simulink model "UAV_USV_Simulator"  (R2017b)
settings: Solver=ode3  StartTime=0.0  StopTime=15  FixedStep=0.01  RelTol=1e-3
PreLoadFcn:
  | addpath(genpath(fileparts(which (bdroot))))
  | 
  | CascadedPID=Simulink.Variant('ControlType==0');
  | InverseKin=Simulink.Variant('ControlType==1');
  | 
  | ControlType = 0;
  | Waypoints = [10 10 ; -10 10 ; -10 -10; 10 -10; 0 0 ];
  | WaypointsX = Waypoints(:,1)'/3;
  | WaypointsY = Waypoints(:,2)'/3;
  | StriderSpeedCmd = 0;
  | 
  | ax=0;
  | ay=0;
  | LandingSchedule = 5;
  | EnableVTOL=1;
  | Psi_cmd = 0;
  | Alt_cmd = 1;
  | 
  | AccRadius =0.5;
  | AppAlt =1;
  | e = 0.1;
PostLoadFcn:
  | addpath(genpath(fileparts(which (bdroot))))
model workspace (MAT data in the model file):
  CD = Simulink.Parameter
  CD.Value = 2.38e-07
  CD.Description = 'Drag/Torque coefficient for the quadcopter rotors'
  CD.DataType = 'auto'
  CD.Dimensions = [1 1]
  CT = Simulink.Parameter
  CT.Value = 9.148e-06
  CT.Description = 'Thrust coefficient for the quadcopter rotors'
  CT.DataType = 'auto'
  CT.Dimensions = [1 1]
  MaxRPM = Simulink.Parameter
  MaxRPM.Value = 5000
  MaxRPM.DataType = 'auto'
  MaxRPM.Dimensions = [1 1]
  RPM2RAD = Simulink.Parameter
  RPM2RAD.Value = 0.10471975512
  RPM2RAD.DataType = 'auto'
  RPM2RAD.Dimensions = [1 1]
  g = Simulink.Parameter
  g.Value = 9.81
  g.DataType = 'auto'
  g.Dimensions = [1 1]
  mass = Simulink.Parameter
  mass.Value = 0.441
  mass.Description = 'Mass of the quadcopter'
  mass.DataType = 'auto'
  mass.Dimensions = [1 1]
undefined symbols (not defined in the file or in its folder): magnitude, sigbuilder_block
libraries: simulink x12, simulink_extras x12, vrlib x5, dsparch4 x1, sharedtransform x1, dspswit3 x1
(part 1 of 2)
settings Model: Creator=Omar Velasco Anrar  LastModifiedBy=omarc
settings DataIOCC: ReturnWorkspaceOutputs=on
settings OptimizationCC: EfficientMapNaN2IntZero=off
settings DebuggingCC: ReadBeforeWriteMsg=DisableAll  WriteAfterWriteMsg=DisableAll  WriteAfterReadMsg=DisableAll  MultiTaskDSMMsg=none
settings HardwareCC: TargetBitPerPointer=64  TargetBitPerSizeT=64  TargetBitPerPtrDiffT=64  TargetLongLongMode=on  TargetIntDivRoundTo=Zero  TargetEndianess=LittleEndian  TargetWordSize=64  TargetHWDeviceType=MATLAB Host  ProdEqTarget=off
settings ModelReferenceCC: UpdateModelReferenceTargets=IfOutOfDate
settings SFSimCC: SFSimEcho=off
settings CodeAppCC: MaxIdLength=128
settings GRTTargetCC: TargetLangStandard=C89/C90 (ANSI)  CombineOutputUpdateFcns=off  GRTInterface=on

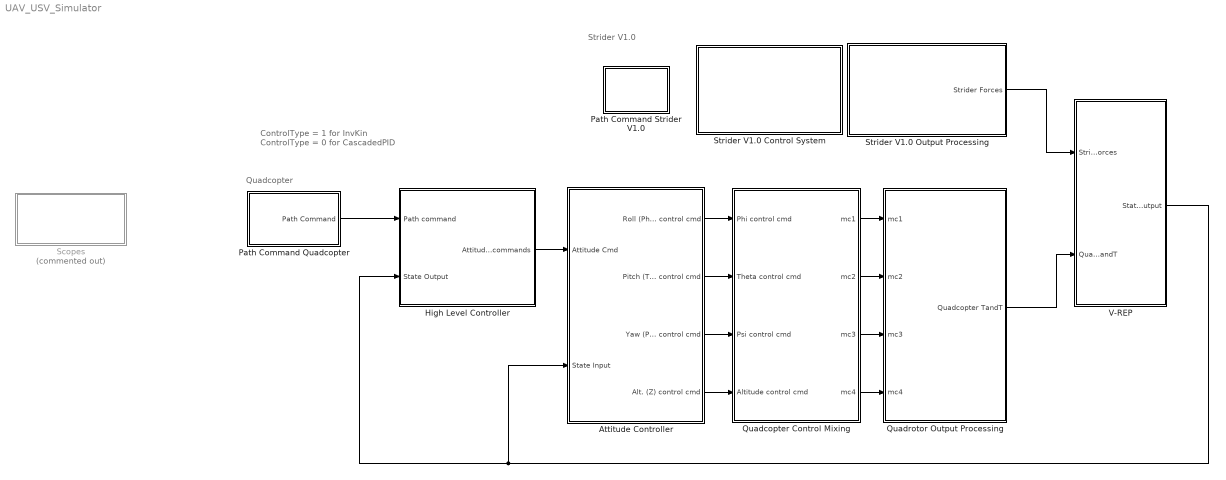
== system UAV_USV_Simulator ==
  note: Quadcopter
  note: Strider V1.0
  note: ControlType = 1 for InvKin
      | ControlType = 0 for CascadedPID
  Attitude Controller : Subsystem
  High Level Controller : Subsystem  Variant=on
  Path Command Quadcopter : Subsystem  Variant=on
  Path Command Strider V1.0 : Subsystem
  Quadcopter Control Mixing : Subsystem
  Quadrotor Output Processing : Subsystem
  "Scopes " : Subsystem  Commented=on
  Strider V1.0 Output Processing : Subsystem
  Strider V1.0 Control System : Subsystem
  V-REP : Subsystem
  wires:
  Quadcopter Control Mixing/4(mc4) -> Quadrotor Output Processing/4(mc4)
  V-REP/1(State Output) -> High Level Controller/2(State Output), Attitude Controller/2(State Input)
  Attitude Controller/4(Alt. (Z) control cmd) -> Quadcopter Control Mixing/4(Altitude control cmd)
  Attitude Controller/2(Pitch (Theta) control cmd) -> Quadcopter Control Mixing/2(Theta control cmd)
  Attitude Controller/3(Yaw (Psi) control cmd) -> Quadcopter Control Mixing/3(Psi control cmd)
  Quadcopter Control Mixing/2(mc2) -> Quadrotor Output Processing/2(mc2)
  Quadcopter Control Mixing/3(mc3) -> Quadrotor Output Processing/3(mc3)
  Quadcopter Control Mixing/1(mc1) -> Quadrotor Output Processing/1(mc1)
  Attitude Controller/1(Roll (Phi) control cmd) -> Quadcopter Control Mixing/1(Phi control cmd)
  High Level Controller/1(Attitude commands) -> Attitude Controller/1(Attitude Cmd)
  Path Command Quadcopter/1(Path Command) -> High Level Controller/1(Path command)
  Quadrotor Output Processing/1("Quadcopter TandT ") -> V-REP/2(Quadcopter TandT)
  Strider V1.0 Output Processing/1(Strider Forces) -> V-REP/1(Strider Forces)

== system UAV_USV_Simulator/Attitude Controller ==
  Attitude Cmd : Inport
  State Input : Inport  Port=2
  Altitude Control : Subsystem
  Bus Selector : BusSelector  OutputSignals=Phi,The,Psi,Z
  Pitch Control : Subsystem
  Roll Control : Subsystem
  Yaw Control : Subsystem
  Roll (Phi) control cmd : Outport
  Pitch (Theta) control cmd : Outport  Port=2
  Yaw (Psi) control cmd : Outport  Port=3
  Alt. (Z) control cmd : Outport  Port=4
  tag scope: Cmds=global
  wires:
  State Input/1 -> Bus Selector/1
  Bus Selector/1 -> Roll Control/2(Phi)  "<Phi>"
  Bus Selector/2 -> Pitch Control/2(Theta)  "<The>"
  Bus Selector/3 -> Yaw Control/2(Psi)  "<Psi>"
  Yaw Control/1(Out1) -> Yaw (Psi) control cmd/1
  Pitch Control/1(Out1) -> Pitch (Theta) control cmd/1
  Roll Control/1(Out1) -> Roll (Phi) control cmd/1
  Attitude Cmd/1 -> Altitude Control/1("Alt_cmd "), Yaw Control/1(Attitude Comand), Pitch Control/1(Attitude Comand), Roll Control/1(Attitude Comand), [Cmds]
  Altitude Control/1(Out) -> Alt. (Z) control cmd/1
  Bus Selector/4 -> Altitude Control/2(Z)  "<Z>"

== system UAV_USV_Simulator/High Level Controller ==
  Path command : Inport
  State Output : Inport  Port=2
  Cascaded PID : Subsystem  VariantControl=CascadedPID
  Inverse kinematics architecture : Subsystem  VariantControl=InverseKin
  Attitude commands : Outport

== system UAV_USV_Simulator/Path Command Quadcopter ==
  "Cascaded PID " : Subsystem  VariantControl=CascadedPID
  Inverse Kinematics : Subsystem  VariantControl=InverseKin
  Path Command : Outport

== system UAV_USV_Simulator/Path Command Strider V1.0 ==
  Constant : Constant  Value=WaypointsX
  Constant1 : Constant  Value=StriderSpeedCmd
  Constant2 : Constant  Value=WaypointsY
  Gain : Gain
  Gain1 : Gain
  tag scope: Speed_command=global, X_waypoints=global, Y_waypoints=global
  wires:
  Constant1/1 -> [Speed_command]
  Gain/1 -> [Y_waypoints]
  Gain1/1 -> [X_waypoints]
  Constant2/1 -> Gain/1
  Constant/1 -> Gain1/1

== system UAV_USV_Simulator/Quadcopter Control Mixing ==
  Phi control cmd : Inport
  Theta control cmd : Inport  Port=2
  Psi control cmd : Inport  Port=3
  Altitude control cmd : Inport  Port=4
  + Config Control Mixing : Subsystem
  mc1 : Outport
  mc2 : Outport  Port=2
  mc3 : Outport  Port=3
  mc4 : Outport  Port=4
  wires:
  Phi control cmd/1 -> + Config Control Mixing/1(Phi rotor cmd)
  Theta control cmd/1 -> + Config Control Mixing/2(Theta rotor cmd)
  Psi control cmd/1 -> + Config Control Mixing/3(Psi rotor cmd)
  Altitude control cmd/1 -> + Config Control Mixing/4(Altitude rotor cmd)
  + Config Control Mixing/1(mc1) -> mc1/1  "mc1"
  + Config Control Mixing/2(mc2) -> mc2/1  "mc2"
  + Config Control Mixing/3(mc3) -> mc3/1  "mc3"
  + Config Control Mixing/4(mc4) -> mc4/1  "mc4"

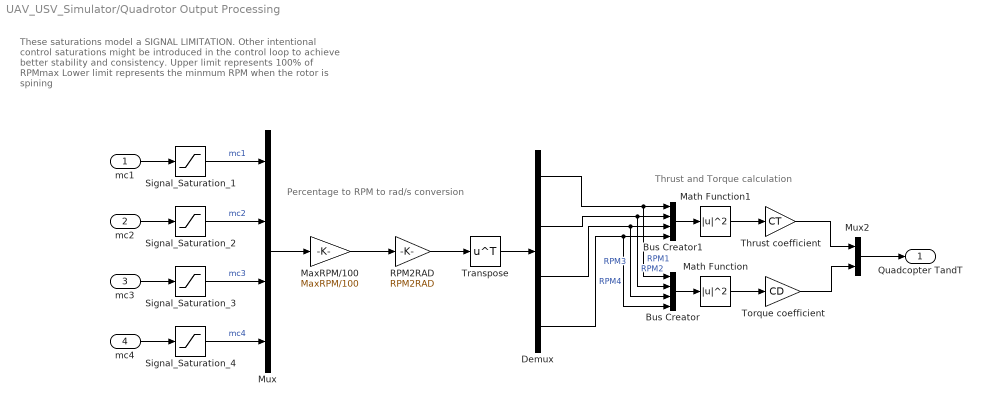
== system UAV_USV_Simulator/Quadrotor Output Processing ==
  note: Percentage to RPM to rad/s conversion
  note: Thrust and Torque calculation
  note: These saturations model a SIGNAL LIMITATION.
      | Other intentional control saturations might be introduced in the
      | control loop to achieve better stability and consistency.
      | Upper limit represents 100% of RPMmax
      | Lower limit represents the minmum RPM when the rotor is spining
  mc1 : Inport
  mc2 : Inport  Port=2
  mc3 : Inport  Port=3
  mc4 : Inport  Port=4
  Bus Creator : BusCreator  Inputs=4
  Bus Creator1 : BusCreator  Inputs=4
  Demux : Demux
  Math Function : Math  Operator=magnitude^2  SaturateOnIntegerOverflow=on
  Math Function1 : Math  Operator=magnitude^2  SaturateOnIntegerOverflow=on
  MaxRPM/100 : Gain  Gain=MaxRPM/100
  Mux : Mux
  Mux2 : Mux  Inputs=2
  RPM2RAD : Gain  Gain=RPM2RAD
  Signal_Saturation_{1..4} (4 alike) : Saturate  UpperLimit=100  LowerLimit=0  ZeroCross=off
  Thrust coefficient : Gain  Gain=CT
  Torque coefficient : Gain  Gain=CD
  Transpose : Math  Operator=transpose  SaturateOnIntegerOverflow=on
  "Quadcopter TandT " : Outport
  wires:
  mc1/1 -> Signal_Saturation_1/1
  mc4/1 -> Signal_Saturation_4/1
  Signal_Saturation_1/1 -> Mux/1  "mc1"
  Signal_Saturation_2/1 -> Mux/2  "mc2"
  Demux/1 -> Bus Creator/1, Bus Creator1/1  "RPM1"
  Demux/2 -> Bus Creator/2, Bus Creator1/2  "RPM2"
  Demux/3 -> Bus Creator/3, Bus Creator1/3  "RPM3"
  Demux/4 -> Bus Creator/4, Bus Creator1/4  "RPM4"
  MaxRPM/100/1 -> RPM2RAD/1
  Mux/1 -> MaxRPM/100/1
  Signal_Saturation_4/1 -> Mux/4  "mc4"
  Bus Creator/1 -> Math Function/1
  Torque coefficient/1 -> Mux2/2
  Thrust coefficient/1 -> Mux2/1
  Math Function/1 -> Torque coefficient/1
  Bus Creator1/1 -> Math Function1/1
  Math Function1/1 -> Thrust coefficient/1
  RPM2RAD/1 -> Transpose/1
  Transpose/1 -> Demux/1
  mc2/1 -> Signal_Saturation_2/1
  mc3/1 -> Signal_Saturation_3/1
  Signal_Saturation_3/1 -> Mux/3  "mc3"
  Mux2/1 -> "Quadcopter TandT "/1

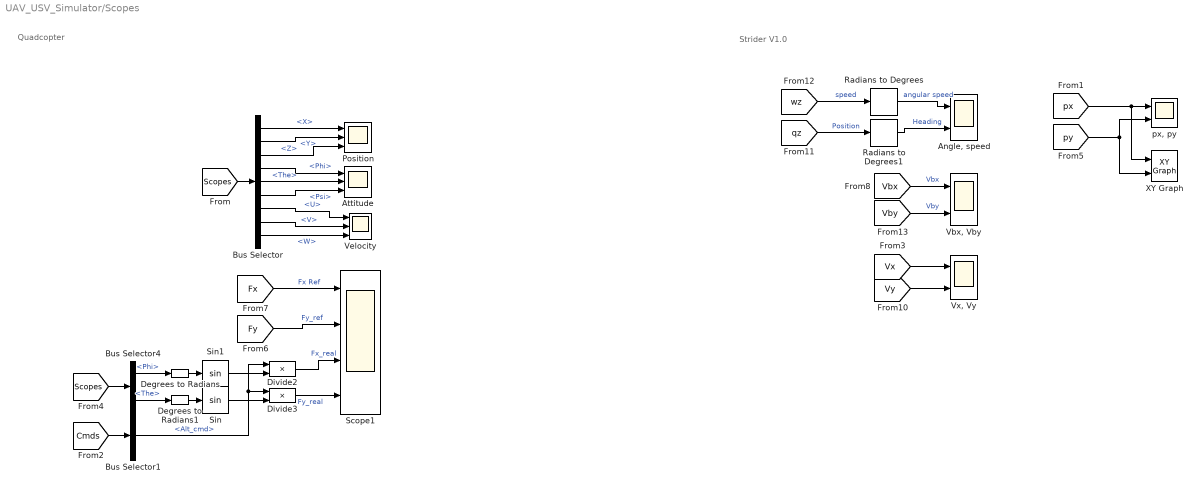
== system UAV_USV_Simulator/Scopes  ==
  note: Strider V1.0
  note: Quadcopter
  "Angle, speed" : Scope  NumInputPorts=2
  Attitude : Scope  NumInputPorts=3
  Bus Selector : BusSelector  OutputSignals=X,Y,Z,Phi,The,Psi,U,V,W
  Bus Selector1 : BusSelector  OutputSignals=Alt_cmd
  Bus Selector4 : BusSelector  OutputSignals=Phi,The
  Degrees to Radians : simulink_extras/Transformations/Degrees to Radians
  Degrees to Radians1 : simulink_extras/Transformations/Degrees to Radians
  Divide2 : Product  Inputs=**
  Divide3 : Product  Inputs=**
  Position : Scope  NumInputPorts=3
  Radians to Degrees : simulink_extras/Transformations/Radians to Degrees
  Radians to Degrees1 : simulink_extras/Transformations/Radians to Degrees
  Scope1 : Scope  NumInputPorts=4
  Sin : Trigonometry
  Sin1 : Trigonometry
  "Vbx, Vby" : Scope  NumInputPorts=2
  Velocity : Scope  NumInputPorts=3
  "Vx, Vy" : Scope  NumInputPorts=2
  XY Graph : simulink/Sinks/XY Graph  xmin=-15  xmax=15  ymin=-15  ymax=15  st=-1
  "px, py" : Scope  NumInputPorts=2
  wires:
  Bus Selector4/1 -> Degrees to Radians/1  "<Phi>"
  Bus Selector4/2 -> Degrees to Radians1/1  "<The>"
  Sin1/1 -> Divide2/2
  [Fy] -> Scope1/2  "Fy_ref"
  [Fx] -> Scope1/1  "Fx Ref"
  Sin/1 -> Divide3/2
  Divide3/1 -> Scope1/4  "Fy_real"
  Divide2/1 -> Scope1/3  "Fx_real"
  Degrees to Radians/1 -> Sin1/1
  Degrees to Radians1/1 -> Sin/1
  [Scopes] -> Bus Selector4/1
  ? -> ?
  Bus Selector/6 -> Attitude/3  "<Psi>"
  Bus Selector/9 -> Velocity/3  "<W>"
  Bus Selector/4 -> Attitude/1  "<Phi>"
  Bus Selector/7 -> Velocity/1  "<U>"
  [Scopes] -> Bus Selector/1
  Bus Selector/5 -> Attitude/2  "<The>"
  Bus Selector/8 -> Velocity/2  "<V>"
  Bus Selector/2 -> Position/2  "<Y>"
  Bus Selector/3 -> Position/3  "<Z>"
  Bus Selector/1 -> Position/1  "<X>"
  [Vx] -> "Vx, Vy"/1
  [Vbx] -> "Vbx, Vby"/1  "Vbx"
  [wz] -> Radians to Degrees/1  "speed"
  [qz] -> Radians to Degrees1/1  "Position"
  Radians to Degrees1/1 -> "Angle, speed"/2  "Heading"
  [Vby] -> "Vbx, Vby"/2  "Vby"
  Radians to Degrees/1 -> "Angle, speed"/1  "angular speed"
  [Vy] -> "Vx, Vy"/2
  [py] -> XY Graph/2, "px, py"/2
  [px] -> XY Graph/1, "px, py"/1
  [Cmds] -> Bus Selector1/1
  Bus Selector1/1 -> Divide3/1, Divide2/1  "<Alt_cmd>"

== system UAV_USV_Simulator/Strider V1.0 Output Processing ==
  Friction forces : Subsystem
  Hydrodinamic forces : Subsystem
  "Inertial to body frame speed " : Subsystem
  Mux3 : Mux  Inputs=6
  Rudder forces1 : Subsystem
  Sum1 : Sum  Inputs=|++
  Strider Forces : Outport
  wires:
  Rudder forces1/2(Y rudder force) -> Mux3/3
  [Thrust_cmd] -> Mux3/1
  Rudder forces1/1(X rudder force) -> Mux3/2
  Mux3/1 -> Strider Forces/1
  Friction forces/2(Ff Y) -> Sum1/1
  Hydrodinamic forces/1(Yhyd) -> Sum1/2
  Friction forces/1(Ff X) -> Mux3/4
  Sum1/1 -> Mux3/5
  Hydrodinamic forces/2(Nhyd) -> Mux3/6

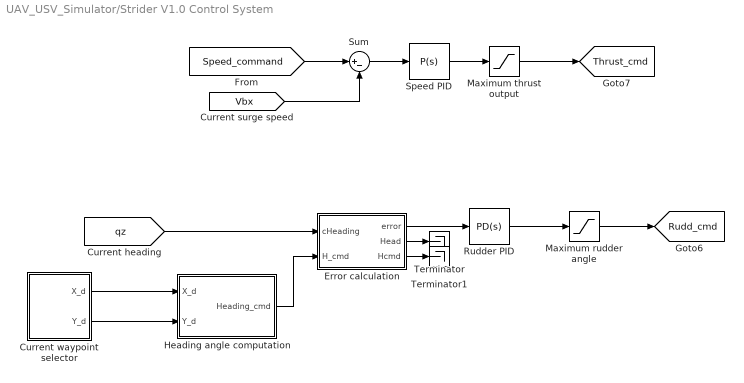
== system UAV_USV_Simulator/Strider V1.0 Control System ==
  Current waypoint selector : Subsystem
  Error calculation : MATLAB Function  TreatAsAtomicUnit=on
  Heading angle computation : Subsystem
  Maximum rudder angle : Saturate  UpperLimit=35*pi/180  LowerLimit=-35*pi/180
  Maximum thrust output : Saturate  UpperLimit=3  LowerLimit=-3
  Rudder PID : simulink/Continuous/PID Controller  Controller=PD  TimeDomain=Continuous-time  SampleTime=-1  IntegratorMethod=Forward Euler  FilterMethod=Forward Euler  Form=Parallel  UseFilter=on  ControllerParametersSource=internal  P=0.5  I=1  D=0.6  N=21.4165136740303  InitialConditionSource=internal  InitialConditionForIntegrator=0  InitialConditionForFilter=0  ExternalReset=none  LimitOutput=off  UpperSaturationLimit=inf  LowerSaturationLimit=-inf  LinearizeAsGain=on  AntiWindupMode=none  Kb=1  TrackingMode=off  Kt=1  PParamMin=[]  PParamMax=[]  IParamMin=[]  IParamMax=[]  DParamMin=[]  DParamMax=[]  NParamMin=[]  NParamMax=[]  KbParamMin=[]  KbParamMax=[]  KtParamMin=[]  KtParamMax=[]  POutMin=[]  POutMax=[]  IOutMin=[]  IOutMax=[]  DOutMin=[]  DOutMax=[]  NOutMin=[]  NOutMax=[]  KbOutMin=[]  KbOutMax=[]  KtOutMin=[]  KtOutMax=[]  IntegratorOutMin=[]  IntegratorOutMax=[]  FilterOutMin=[]  FilterOutMax=[]  SumOutMin=[]  SumOutMax=[]  SumI1OutMin=[]  SumI1OutMax=[]  SumI2OutMin=[]  SumI2OutMax=[]  SumI3OutMin=[]  SumI3OutMax=[]  SumDOutMin=[]  SumDOutMax=[]  SaturationOutMin=[]  SaturationOutMax=[]  IntegratorContinuousStateAttributes=''  IntegratorStateMustResolveToSignalObject=off  IntegratorRTWStateStorageClass=Auto  FilterContinuousStateAttributes=''  FilterStateMustResolveToSignalObject=off  FilterRTWStateStorageClass=Auto  DifferentiatorICPrevScaledInput=0  DifferentiatorOutMin=[]  DifferentiatorOutMax=[]  InitialConditionSetting=State (most efficient)  FilterDiffOutCoefMin=[]  FilterDiffOutCoefMax=[]  SumDenOutMin=[]  SumDenOutMax=[]  SumNumOutMin=[]  SumNumOutMax=[]  ReciprocalOutMin=[]  ReciprocalOutMax=[]  DivideOutMin=[]  DivideOutMax=[]  TunerSelectOption=Transfer Function Based (PID Tuner App)
  "Speed PID " : simulink/Continuous/PID Controller  Controller=P  TimeDomain=Continuous-time  SampleTime=-1  IntegratorMethod=Forward Euler  FilterMethod=Forward Euler  Form=Parallel  UseFilter=on  ControllerParametersSource=internal  P=82.65  I=27.6098096977436  D=0  N=100  InitialConditionSource=internal  InitialConditionForIntegrator=0  InitialConditionForFilter=0  ExternalReset=none  LimitOutput=off  UpperSaturationLimit=inf  LowerSaturationLimit=-inf  LinearizeAsGain=on  AntiWindupMode=none  Kb=1  TrackingMode=off  Kt=1  PParamMin=[]  PParamMax=[]  IParamMin=[]  IParamMax=[]  DParamMin=[]  DParamMax=[]  NParamMin=[]  NParamMax=[]  KbParamMin=[]  KbParamMax=[]  KtParamMin=[]  KtParamMax=[]  POutMin=[]  POutMax=[]  IOutMin=[]  IOutMax=[]  DOutMin=[]  DOutMax=[]  NOutMin=[]  NOutMax=[]  KbOutMin=[]  KbOutMax=[]  KtOutMin=[]  KtOutMax=[]  IntegratorOutMin=[]  IntegratorOutMax=[]  FilterOutMin=[]  FilterOutMax=[]  SumOutMin=[]  SumOutMax=[]  SumI1OutMin=[]  SumI1OutMax=[]  SumI2OutMin=[]  SumI2OutMax=[]  SumI3OutMin=[]  SumI3OutMax=[]  SumDOutMin=[]  SumDOutMax=[]  SaturationOutMin=[]  SaturationOutMax=[]  IntegratorContinuousStateAttributes=''  IntegratorStateMustResolveToSignalObject=off  IntegratorRTWStateStorageClass=Auto  FilterContinuousStateAttributes=''  FilterStateMustResolveToSignalObject=off  FilterRTWStateStorageClass=Auto  DifferentiatorICPrevScaledInput=0  DifferentiatorOutMin=[]  DifferentiatorOutMax=[]  InitialConditionSetting=State (most efficient)  FilterDiffOutCoefMin=[]  FilterDiffOutCoefMax=[]  SumDenOutMin=[]  SumDenOutMax=[]  SumNumOutMin=[]  SumNumOutMax=[]  ReciprocalOutMin=[]  ReciprocalOutMax=[]  DivideOutMin=[]  DivideOutMax=[]  TunerSelectOption=Transfer Function Based (PID Tuner App)
  Sum : Sum  Inputs=|+-
  Terminator : Terminator
  Terminator1 : Terminator
  tag scope: Rudd_cmd=global, Thrust_cmd=global
  wires:
  "Speed PID "/1 -> Maximum thrust output/1
  Error calculation/1(error) -> Rudder PID/1
  [Speed_command] -> Sum/1
  Sum/1 -> "Speed PID "/1
  Maximum rudder angle/1 -> [Rudd_cmd]
  Rudder PID/1 -> Maximum rudder angle/1
  [Vbx] -> Sum/2
  Maximum thrust output/1 -> [Thrust_cmd]
  Heading angle computation/1(Heading_cmd) -> Error calculation/2(H_cmd)
  [qz] -> Error calculation/1(cHeading)
  Current waypoint selector/1(X_d) -> Heading angle computation/1(X_d)
  Current waypoint selector/2(Y_d) -> Heading angle computation/2(Y_d)
  Error calculation/2(Head) -> Terminator/1
  Error calculation/3(Hcmd) -> Terminator1/1

== system UAV_USV_Simulator/V-REP ==
  Strider Forces : Inport
  Quadcopter TandT : Inport  Port=2
  Mux1 : Mux  Inputs=2
  Subsystem2 : Subsystem
  Terminator : Terminator
  To V-REP1 : S-Function  FunctionName=Vrep_API_Script  SFunctionDeploymentMode=off  EnableBusSupport=off
  State Output : Outport
  tag scope: Scopes=global
  wires:
  Quadcopter TandT/1 -> Mux1/1
  Mux1/1 -> To V-REP1/1
  Strider Forces/1 -> Mux1/2
  To V-REP1/1 -> Subsystem2/1(V-REP array)
  Subsystem2/1(State Output) -> [Scopes], State Output/1
  Subsystem2/2(State Output Str) -> Terminator/1

== system UAV_USV_Simulator/Attitude Controller/Altitude Control ==
  "Alt_cmd " : Inport
  Z : Inport  Port=2
  Altitude controller : Subsystem  Variant=on
  Out : Outport
  wires:
  Altitude controller/1(Out) -> Out/1
  Z/1 -> Altitude controller/2(Z)
  "Alt_cmd "/1 -> Altitude controller/1(Alt_cmd)

== system UAV_USV_Simulator/Attitude Controller/Pitch Control ==
  Attitude Comand : Inport
  Theta : Inport  Port=2
  Bus Selector : BusSelector  OutputSignals=The_cmd
  PID Controller1 : simulink/Continuous/PID Controller  Controller=PID  TimeDomain=Continuous-time  SampleTime=-1  IntegratorMethod=Forward Euler  FilterMethod=Forward Euler  Form=Parallel  UseFilter=on  ControllerParametersSource=internal  P=0.3217336  I=0.4324  D=0.0583122  N=100  InitialConditionSource=internal  InitialConditionForIntegrator=0  InitialConditionForFilter=0  ExternalReset=none  LimitOutput=on  UpperSaturationLimit=20  LowerSaturationLimit=-20  LinearizeAsGain=on  AntiWindupMode=none  Kb=1  TrackingMode=off  Kt=1  PParamMin=[]  PParamMax=[]  IParamMin=[]  IParamMax=[]  DParamMin=[]  DParamMax=[]  NParamMin=[]  NParamMax=[]  KbParamMin=[]  KbParamMax=[]  KtParamMin=[]  KtParamMax=[]  POutMin=[]  POutMax=[]  IOutMin=[]  IOutMax=[]  DOutMin=[]  DOutMax=[]  NOutMin=[]  NOutMax=[]  KbOutMin=[]  KbOutMax=[]  KtOutMin=[]  KtOutMax=[]  IntegratorOutMin=[]  IntegratorOutMax=[]  FilterOutMin=[]  FilterOutMax=[]  SumOutMin=[]  SumOutMax=[]  SumI1OutMin=[]  SumI1OutMax=[]  SumI2OutMin=[]  SumI2OutMax=[]  SumI3OutMin=[]  SumI3OutMax=[]  SumDOutMin=[]  SumDOutMax=[]  SaturationOutMin=[]  SaturationOutMax=[]  IntegratorContinuousStateAttributes=''  IntegratorStateMustResolveToSignalObject=off  IntegratorRTWStateStorageClass=Auto  FilterContinuousStateAttributes=''  FilterStateMustResolveToSignalObject=off  FilterRTWStateStorageClass=Auto  DifferentiatorICPrevScaledInput=0  DifferentiatorOutMin=[]  DifferentiatorOutMax=[]  InitialConditionSetting=State (most efficient)  FilterDiffOutCoefMin=[]  FilterDiffOutCoefMax=[]  SumDenOutMin=[]  SumDenOutMax=[]  SumNumOutMin=[]  SumNumOutMax=[]  ReciprocalOutMin=[]  ReciprocalOutMax=[]  DivideOutMin=[]  DivideOutMax=[]  TunerSelectOption=Transfer Function Based (PID Tuner App)
  Sum : Sum  Inputs=|+-
  Out1 : Outport
  wires:
  Attitude Comand/1 -> Bus Selector/1
  Theta/1 -> Sum/2
  Bus Selector/1 -> Sum/1  "<The_cmd>"
  PID Controller1/1 -> Out1/1
  Sum/1 -> PID Controller1/1

== system UAV_USV_Simulator/Attitude Controller/Roll Control ==
  Attitude Comand : Inport
  Phi : Inport  Port=2
  Bus Selector : BusSelector  OutputSignals=Phi_cmd
  PID Controller1 : simulink/Continuous/PID Controller  Controller=PID  TimeDomain=Continuous-time  SampleTime=-1  IntegratorMethod=Forward Euler  FilterMethod=Forward Euler  Form=Parallel  UseFilter=on  ControllerParametersSource=internal  P=0.3217  I=0.4324  D=0.0583  N=100  InitialConditionSource=internal  InitialConditionForIntegrator=0.18  InitialConditionForFilter=0  ExternalReset=none  LimitOutput=on  UpperSaturationLimit=20  LowerSaturationLimit=-20  LinearizeAsGain=on  AntiWindupMode=none  Kb=1  TrackingMode=off  Kt=1  PParamMin=[]  PParamMax=[]  IParamMin=[]  IParamMax=[]  DParamMin=[]  DParamMax=[]  NParamMin=[]  NParamMax=[]  KbParamMin=[]  KbParamMax=[]  KtParamMin=[]  KtParamMax=[]  POutMin=[]  POutMax=[]  IOutMin=[]  IOutMax=[]  DOutMin=[]  DOutMax=[]  NOutMin=[]  NOutMax=[]  KbOutMin=[]  KbOutMax=[]  KtOutMin=[]  KtOutMax=[]  IntegratorOutMin=[]  IntegratorOutMax=[]  FilterOutMin=[]  FilterOutMax=[]  SumOutMin=[]  SumOutMax=[]  SumI1OutMin=[]  SumI1OutMax=[]  SumI2OutMin=[]  SumI2OutMax=[]  SumI3OutMin=[]  SumI3OutMax=[]  SumDOutMin=[]  SumDOutMax=[]  SaturationOutMin=[]  SaturationOutMax=[]  IntegratorContinuousStateAttributes=''  IntegratorStateMustResolveToSignalObject=off  IntegratorRTWStateStorageClass=Auto  FilterContinuousStateAttributes=''  FilterStateMustResolveToSignalObject=off  FilterRTWStateStorageClass=Auto  DifferentiatorICPrevScaledInput=0  DifferentiatorOutMin=[]  DifferentiatorOutMax=[]  InitialConditionSetting=State (most efficient)  FilterDiffOutCoefMin=[]  FilterDiffOutCoefMax=[]  SumDenOutMin=[]  SumDenOutMax=[]  SumNumOutMin=[]  SumNumOutMax=[]  ReciprocalOutMin=[]  ReciprocalOutMax=[]  DivideOutMin=[]  DivideOutMax=[]  TunerSelectOption=Transfer Function Based (PID Tuner App)
  Sum : Sum  Inputs=|+-
  Out1 : Outport
  wires:
  Attitude Comand/1 -> Bus Selector/1
  Phi/1 -> Sum/2
  Sum/1 -> PID Controller1/1
  Bus Selector/1 -> Sum/1  "<Phi_cmd>"
  PID Controller1/1 -> Out1/1

== system UAV_USV_Simulator/Attitude Controller/Yaw Control ==
  Attitude Comand : Inport
  Psi : Inport  Port=2
  Bus Selector : BusSelector  OutputSignals=Psi_cmd
  PID Controller : simulink/Continuous/PID Controller  Controller=PID  TimeDomain=Continuous-time  SampleTime=-1  IntegratorMethod=Forward Euler  FilterMethod=Forward Euler  Form=Parallel  UseFilter=on  ControllerParametersSource=internal  P=0.665668467901894  I=0.340149010656045  D=0.313800354221384  N=96.4244783671056  InitialConditionSource=internal  InitialConditionForIntegrator=0.0095  InitialConditionForFilter=0  ExternalReset=none  LimitOutput=on  UpperSaturationLimit=10  LowerSaturationLimit=-10  LinearizeAsGain=on  AntiWindupMode=clamping  Kb=1  TrackingMode=off  Kt=1  PParamMin=[]  PParamMax=[]  IParamMin=[]  IParamMax=[]  DParamMin=[]  DParamMax=[]  NParamMin=[]  NParamMax=[]  KbParamMin=[]  KbParamMax=[]  KtParamMin=[]  KtParamMax=[]  POutMin=[]  POutMax=[]  IOutMin=[]  IOutMax=[]  DOutMin=[]  DOutMax=[]  NOutMin=[]  NOutMax=[]  KbOutMin=[]  KbOutMax=[]  KtOutMin=[]  KtOutMax=[]  IntegratorOutMin=[]  IntegratorOutMax=[]  FilterOutMin=[]  FilterOutMax=[]  SumOutMin=[]  SumOutMax=[]  SumI1OutMin=[]  SumI1OutMax=[]  SumI2OutMin=[]  SumI2OutMax=[]  SumI3OutMin=[]  SumI3OutMax=[]  SumDOutMin=[]  SumDOutMax=[]  SaturationOutMin=[]  SaturationOutMax=[]  IntegratorContinuousStateAttributes=''  IntegratorStateMustResolveToSignalObject=off  IntegratorRTWStateStorageClass=Auto  FilterContinuousStateAttributes=''  FilterStateMustResolveToSignalObject=off  FilterRTWStateStorageClass=Auto  DifferentiatorICPrevScaledInput=0  DifferentiatorOutMin=[]  DifferentiatorOutMax=[]  InitialConditionSetting=State (most efficient)  FilterDiffOutCoefMin=[]  FilterDiffOutCoefMax=[]  SumDenOutMin=[]  SumDenOutMax=[]  SumNumOutMin=[]  SumNumOutMax=[]  ReciprocalOutMin=[]  ReciprocalOutMax=[]  DivideOutMin=[]  DivideOutMax=[]  TunerSelectOption=Transfer Function Based (PID Tuner App)
  Sum : Sum  Inputs=|+-
  Out1 : Outport
  wires:
  Attitude Comand/1 -> Bus Selector/1
  Sum/1 -> PID Controller/1
  Bus Selector/1 -> Sum/1  "<Psi_cmd>"
  Psi/1 -> Sum/2
  PID Controller/1 -> Out1/1

== system UAV_USV_Simulator/High Level Controller/Cascaded PID ==
  Path command : Inport
  State Output : Inport  Port=2
  Position Controller : Subsystem
  Velocity Controller : Subsystem
  Attitude commands : Outport
  wires:
  State Output/1 -> Velocity Controller/4("State input "), Position Controller/2(State input)
  Position Controller/3(Path_cmd) -> Velocity Controller/3(Path command)
  Velocity Controller/1(Attitude Cmd) -> Attitude commands/1
  Position Controller/1(Vy_cmd) -> Velocity Controller/1(Vy_cmd)
  Position Controller/2(Vx_cmd) -> Velocity Controller/2(Vx_cmd)
  Path command/1 -> Position Controller/1(Path Command)

== system UAV_USV_Simulator/High Level Controller/Inverse kinematics architecture ==
  Path command : Inport
  "State Output " : Inport  Port=2
  Altitude Control : Subsystem
  Bus Creator1 : BusCreator  Inputs=4
  Bus Selector : BusSelector  OutputSignals=Psi_cmd,ax,ay
  Gain : Gain  Gain=mass
  Gain1 : Gain  Gain=mass
  Thrust and angle calculation3 : Subsystem
  Attitude commands : Outport
  wires:
  "State Output "/1 -> Altitude Control/2(Z)
  Bus Selector/2 -> Gain/1  "<ax>"
  Bus Selector/3 -> Gain1/1  "<ay>"
  Bus Selector/1 -> Thrust and angle calculation3/1(Yaw angle)  "<Psi_cmd>"
  Altitude Control/1(Out1) -> Thrust and angle calculation3/4(Fz)  "Alt_cmd"
  Thrust and angle calculation3/3(Psi_cmd) -> Bus Creator1/3  "Psi_cmd"
  Path command/1 -> Bus Selector/1, Altitude Control/1(Attitude Comand)
  Bus Creator1/1 -> Attitude commands/1
  Thrust and angle calculation3/2(The_cmd) -> Bus Creator1/2  "The_cmd"
  Thrust and angle calculation3/4(Thrust value) -> Bus Creator1/4  "Alt_cmd"
  Thrust and angle calculation3/1(Phi_cmd) -> Bus Creator1/1  "Phi_cmd"
  Gain/1 -> Thrust and angle calculation3/2(Fx)  "Fx"
  Gain1/1 -> Thrust and angle calculation3/3(Fy)  "Fy"

== system UAV_USV_Simulator/Path Command Quadcopter/Cascaded PID  ==
  Bus Creator : BusCreator  Inputs=4
  Constant3 : Constant  Value=Psi_cmd
  VTOL Algorithm : Subsystem
  Path Command : Outport
  wires:
  Constant3/1 -> Bus Creator/4  "Psi_cmd"
  Bus Creator/1 -> Path Command/1
  VTOL Algorithm/1(Altitude cmd) -> Bus Creator/3  "Alt_cmd"
  [px] -> Bus Creator/1  "X_cmd"
  [py] -> Bus Creator/2  "Y_cmd"

== system UAV_USV_Simulator/Path Command Quadcopter/Inverse Kinematics ==
  Bus Creator : BusCreator  Inputs=4
  Constant : Constant  Value=Alt_cmd
  Constant1 : Constant  Value=Psi_cmd
  Constant2 : Constant  Commented=on  Value=ax
  Constant3 : Constant  Commented=on  Value=ay
  From Workspace : FromWorkspace  VariableName=ax  SampleTime=0.01  OutputAfterFinalValue=Setting to zero
  From Workspace1 : FromWorkspace  VariableName=ay  SampleTime=0.01  OutputAfterFinalValue=Setting to zero
  Gain1 : Gain
  Gain2 : Gain
  Signal Builder : Subsystem  Tag=STV Subsys  LoadFcn=sigbuilder_block('load');  StartFcn=sigbuilder_block('start');  StopFcn=sigbuilder_block('stop');  ClipboardFcn=sigbuilder_block('clipboard');  mask(Sigbuilder block){tuvar=[0:10]}
      mask help: Simulink:masks:SigbuilderBlock_MD
      mask init:
      | if ~strcmp(get_param(bdroot(gcbh),'SimulationStatus'),'stopped') tuvar = sigbuilder_block('maskInit'); end
      settings: CopyFcn=sigbuilder_block('copy');  DeleteFcn=sigbuilder_block('delete');  ModelCloseFcn=sigbuilder_block('modelClose');  PreSaveFcn=sigbuilder_block('preSave');  PauseFcn=sigbuilder_block('pause');  ContinueFcn=sigbuilder_block('continue');  NameChangeFcn=sigbuilder_block('namechange');  OpenFcn=sigbuilder_block('open',[298.5 220.5 550.5 386.25 ]);  CloseFcn=sigbuilder_block('close');
      mask Display: plot(0, 0, 100, 100,[2, 2, 32, 32, 2], [68, 8, 8, 68, 68],[32, 2], [38, 38], [32, 19, 2],[53, 60, 44], [32, 17, 17, 2],[16, 16, 31, 31]);txt = getActiveGroup(gcbh);text(2, 100, txt,'verticalAlignment', 'top');
  Path Command : Outport
  wires:
  Bus Creator/1 -> Path Command/1
  Gain1/1 -> Bus Creator/2  "ay"
  Constant1/1 -> Bus Creator/3  "Psi_cmd"
  Gain2/1 -> Bus Creator/1  "ax"
  Constant/1 -> Bus Creator/4  "Alt_cmd"
  From Workspace/1 -> Gain2/1
  From Workspace1/1 -> Gain1/1

== system UAV_USV_Simulator/Quadcopter Control Mixing/+ Config Control Mixing ==
  note: mc2 = Alt_cor + Psi_cor + Phi_cor
  note: Control Mixing
  note: mc4 = Alt_cor + Psi_cor - Phi_cor
  note: mc3 = Alt_cor - Psi_cor -The_cor
  note: mc1 = Alt_cor -Psi_cor + The_cor
  Phi rotor cmd : Inport
  Theta rotor cmd : Inport  Port=2
  Psi rotor cmd : Inport  Port=3
  Altitude rotor cmd : Inport  Port=4
  Sum1 : Sum  Inputs=|++
  Sum11 : Sum  Inputs=-+|
  Sum2 : Sum  Inputs=|+-
  Sum3 : Sum  Inputs=-+|
  Sum4 : Sum  Inputs=++|
  Sum8 : Sum  Inputs=|++
  mc1 : Outport
  mc2 : Outport  Port=2
  mc3 : Outport  Port=3
  mc4 : Outport  Port=4
  wires:
  Theta rotor cmd/1 -> Sum1/2, Sum3/1
  Altitude rotor cmd/1 -> Sum2/1, Sum4/2
  Sum2/1 -> Sum3/2, Sum1/1
  Psi rotor cmd/1 -> Sum4/1, Sum2/2
  Sum4/1 -> Sum11/2, Sum8/1
  Phi rotor cmd/1 -> Sum8/2, Sum11/1
  Sum1/1 -> mc1/1
  Sum3/1 -> mc3/1
  Sum8/1 -> mc2/1
  Sum11/1 -> mc4/1

== system UAV_USV_Simulator/Strider V1.0 Output Processing/Friction forces ==
  Gain1 : Gain  Gain=-0.1
  Gain2 : Gain  Gain=-0.1
  Math Function : Math  Operator=magnitude^2  SaturateOnIntegerOverflow=on
  Math Function1 : Math  Operator=magnitude^2  SaturateOnIntegerOverflow=on
  Product2 : Product  Inputs=**
  Product3 : Product  Inputs=**
  Sign : Signum
  Sign1 : Signum
  Ff X : Outport
  Ff Y : Outport  Port=2
  wires:
  Gain1/1 -> Ff Y/1
  Gain2/1 -> Ff X/1
  Product2/1 -> Gain2/1
  Math Function/1 -> Product2/2
  Sign/1 -> Product2/1
  [Vbx] -> Sign/1, Math Function/1
  Product3/1 -> Gain1/1
  Sign1/1 -> Product3/1
  Math Function1/1 -> Product3/2
  [Vby] -> Sign1/1, Math Function1/1

== system UAV_USV_Simulator/Strider V1.0 Output Processing/Hydrodinamic forces ==
  Gain : Gain  Gain=2
  Gain1 : Gain  Gain=-3.899501881
  Gain2 : Gain  Gain=1.774273356
  Gain3 : Gain  Gain=-1.774273356
  Gain4 : Gain  Gain=-0.807294377
  Gain7 : Gain  Gain=2
  Sum : Sum  Inputs=|++
  Sum1 : Sum  Inputs=|++
  Yhyd : Outport
  Nhyd : Outport  Port=2
  wires:
  Gain1/1 -> Sum/1
  Gain3/1 -> Sum1/1
  Gain2/1 -> Sum/2
  [Vby] -> Gain3/1, Gain1/1
  Gain/1 -> Yhyd/1  "Yhyd"
  [wz] -> Gain4/1, Gain2/1
  Gain7/1 -> Nhyd/1  "Nhyd"
  Gain4/1 -> Sum1/2
  Sum/1 -> Gain/1  "Yhyd"
  Sum1/1 -> Gain7/1  "Nhyd"

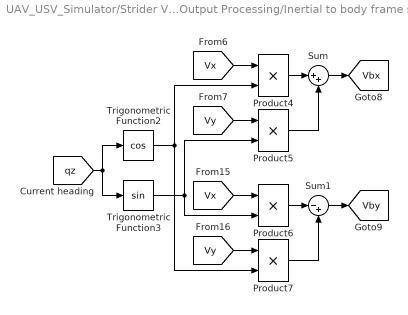
== system UAV_USV_Simulator/Strider V1.0 Output Processing/Inertial to body frame speed  ==
  Product{4..7} (4 alike) : Product  Inputs=**
  Sum : Sum  Inputs=|++
  Sum1 : Sum  Inputs=|-+
  Trigonometric Function2 : Trigonometry  Operator=cos
  Trigonometric Function3 : Trigonometry
  tag scope: Vbx=global, Vby=global
  wires:
  [Vy] -> Product5/1
  [qz] -> Trigonometric Function3/1, Trigonometric Function2/1
  Sum/1 -> [Vbx]
  Sum1/1 -> [Vby]
  Product7/1 -> Sum1/2
  Product6/1 -> Sum1/1
  [Vx] -> Product6/1
  [Vy] -> Product7/1
  Trigonometric Function3/1 -> Product5/2, Product6/2
  Trigonometric Function2/1 -> Product4/2, Product7/2
  [Vx] -> Product4/1
  Product4/1 -> Sum/1
  Product5/1 -> Sum/2

== system UAV_USV_Simulator/Strider V1.0 Output Processing/Rudder forces1 ==
  Gain : Gain  Gain=-1
  Product : Product  Inputs=**
  Product1 : Product  Inputs=**
  Trigonometric Function : Trigonometry
  Trigonometric Function1 : Trigonometry  Operator=cos
  "rudder Force " : Subsystem
  X rudder force : Outport
  Y rudder force : Outport  Port=2
  wires:
  Trigonometric Function/1 -> Product/2
  "rudder Force "/1(Rudder force) -> Product1/2, Product/1
  [Rudd_cmd] -> Trigonometric Function1/1, Trigonometric Function/1
  Product1/1 -> Y rudder force/1  "Yrudder force"
  Gain/1 -> X rudder force/1  "Xrudder force"
  Trigonometric Function1/1 -> Product1/1
  Product/1 -> Gain/1

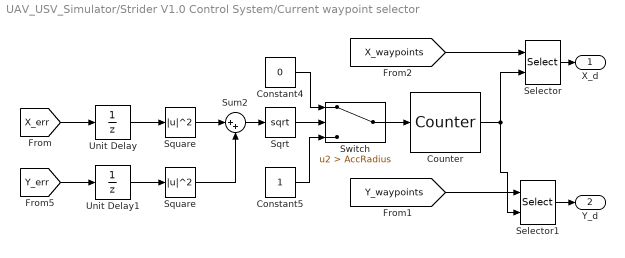
== system UAV_USV_Simulator/Strider V1.0 Control System/Current waypoint selector ==
  Constant4 : Constant  Value=0
  Constant5 : Constant
  Counter : dspswit3/Counter  Direction=Up  CountEvent=Rising edge  CounterSize=User defined  MaxCount=size(WaypointsX,2)  InitialCount=1  Output=Count  HitValue=32  ResetInput=off  SamplesPerFrame=1  Ts=1  CntDtype=uint32  HitDtype=Logical
  Selector : Selector  IndexOptions=Index vector (port)  Indices=[1 3]  OutputSizes=1
  Selector1 : Selector  IndexOptions=Index vector (port)  Indices=[1 3]  OutputSizes=1
  Sqrt : Sqrt  SaturateOnIntegerOverflow=on
  Square : Math  Operator=magnitude^2  SaturateOnIntegerOverflow=on
  "Square " : Math  Operator=magnitude^2  SaturateOnIntegerOverflow=on
  Sum2 : Sum  Inputs=|++
  Switch : Switch  Criteria=u2 > Threshold  Threshold=AccRadius
  Unit Delay : UnitDelay  SampleTime=-1
  Unit Delay1 : UnitDelay  SampleTime=-1
  X_d : Outport
  Y_d : Outport  Port=2
  wires:
  Square/1 -> Sum2/1
  [Y_err] -> Unit Delay1/1
  Selector/1 -> X_d/1
  Constant4/1 -> Switch/1
  Sum2/1 -> Sqrt/1
  Counter/1 -> Selector/2, Selector1/2
  Sqrt/1 -> Switch/2
  Switch/1 -> Counter/1
  [X_err] -> Unit Delay/1
  "Square "/1 -> Sum2/2
  Selector1/1 -> Y_d/1
  Constant5/1 -> Switch/3
  [Y_waypoints] -> Selector1/1
  [X_waypoints] -> Selector/1
  Unit Delay/1 -> Square/1
  Unit Delay1/1 -> "Square "/1

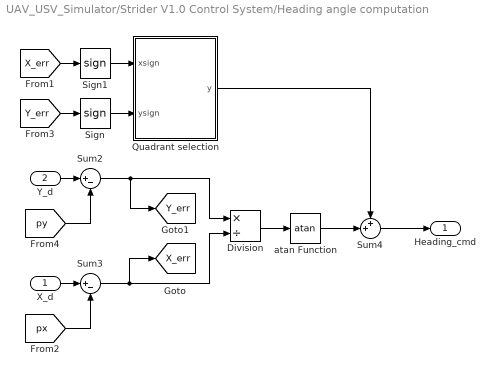
== system UAV_USV_Simulator/Strider V1.0 Control System/Heading angle computation ==
  X_d : Inport
  Y_d : Inport  Port=2
  Division : Product  Inputs=*/
  Quadrant selection : MATLAB Function  TreatAsAtomicUnit=on
  Sign : Signum
  Sign1 : Signum
  Sum2 : Sum  Inputs=|+-
  Sum3 : Sum  Inputs=|+-
  Sum4 : Sum  Inputs=++|
  atan Function : Trigonometry  Operator=atan
  Heading_cmd : Outport
  tag scope: X_err=global, Y_err=global
  wires:
  [py] -> Sum2/2
  Division/1 -> atan Function/1
  X_d/1 -> Sum3/1
  [px] -> Sum3/2
  atan Function/1 -> Sum4/2
  Y_d/1 -> Sum2/1
  Quadrant selection/1(y) -> Sum4/1
  Sign1/1 -> Quadrant selection/1(xsign)
  Sign/1 -> Quadrant selection/2(ysign)
  Sum3/1 -> [X_err], Division/2
  Sum2/1 -> [Y_err], Division/1
  [X_err] -> Sign1/1
  [Y_err] -> Sign/1
  Sum4/1 -> Heading_cmd/1

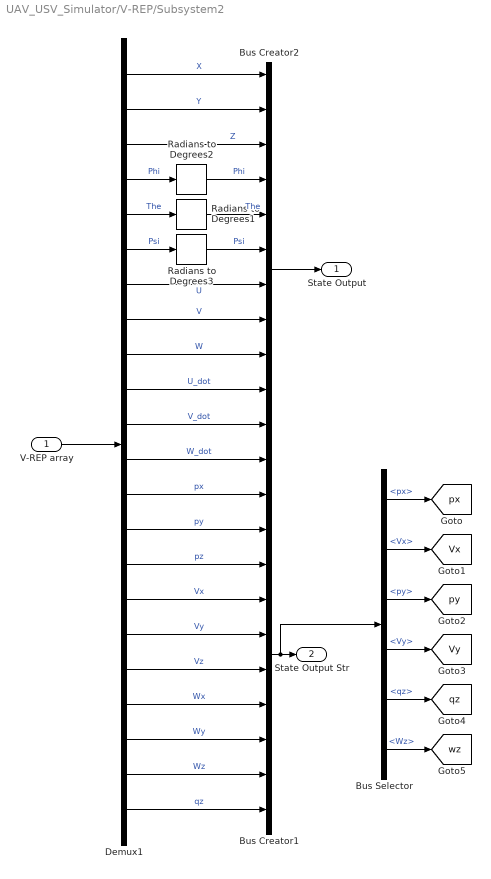
== system UAV_USV_Simulator/V-REP/Subsystem2 ==
  V-REP array : Inport
  Bus Creator1 : BusCreator  Inputs=10
  Bus Creator2 : BusCreator  Inputs=12
  Bus Selector : BusSelector  OutputSignals=px,Vx,py,Vy,qz,Wz
  Demux1 : Demux  Outputs=22
  Radians to Degrees1 : simulink_extras/Transformations/Radians to Degrees
  Radians to Degrees2 : simulink_extras/Transformations/Radians to Degrees
  Radians to Degrees3 : simulink_extras/Transformations/Radians to Degrees
  State Output : Outport
  State Output Str : Outport  Port=2
  tag scope: Vx=global, Vy=global, px=global, py=global, qz=global, wz=global
  wires:
  Demux1/3 -> Bus Creator2/3  "Z"
  Radians to Degrees2/1 -> Bus Creator2/4  "Phi"
  Radians to Degrees1/1 -> Bus Creator2/5  "The"
  Radians to Degrees3/1 -> Bus Creator2/6  "Psi"
  Demux1/7 -> Bus Creator2/7  "U"
  Demux1/2 -> Bus Creator2/2  "Y"
  Demux1/1 -> Bus Creator2/1  "X"
  Demux1/9 -> Bus Creator2/9  "W"
  Demux1/6 -> Radians to Degrees3/1  "Psi"
  Demux1/11 -> Bus Creator2/11  "V_dot"
  Demux1/12 -> Bus Creator2/12  "W_dot"
  V-REP array/1 -> Demux1/1
  Demux1/8 -> Bus Creator2/8  "V"
  Demux1/10 -> Bus Creator2/10  "U_dot"
  Demux1/5 -> Radians to Degrees1/1  "The"
  Demux1/4 -> Radians to Degrees2/1  "Phi"
  Bus Creator2/1 -> State Output/1
  Bus Creator1/1 -> Bus Selector/1, State Output Str/1
  Demux1/13 -> Bus Creator1/1  "px"
  Demux1/14 -> Bus Creator1/2  "py"
  Demux1/15 -> Bus Creator1/3  "pz"
  Demux1/16 -> Bus Creator1/4  "Vx"
  Demux1/17 -> Bus Creator1/5  "Vy"
  Demux1/18 -> Bus Creator1/6  "Vz"
  Demux1/19 -> Bus Creator1/7  "Wx"
  Demux1/20 -> Bus Creator1/8  "Wy"
  Demux1/21 -> Bus Creator1/9  "Wz"
  Demux1/22 -> Bus Creator1/10  "qz"
  Bus Selector/1 -> [px]  "<px>"
  Bus Selector/2 -> [Vx]  "<Vx>"
  Bus Selector/4 -> [Vy]  "<Vy>"
  Bus Selector/3 -> [py]  "<py>"
  Bus Selector/5 -> [qz]  "<qz>"
  Bus Selector/6 -> [wz]  "<Wz>"

== system UAV_USV_Simulator/Attitude Controller/Altitude Control/Altitude controller ==
  Alt_cmd : Inport
  Z : Inport  Port=2
  Altitude PID Control : Subsystem  VariantControl=CascadedPID
  Inverse Kinematics Altitude : Subsystem  VariantControl=InverseKin
  Out : Outport

== system UAV_USV_Simulator/High Level Controller/Cascaded PID/Position Controller ==
  Path Command : Inport
  State input : Inport  Port=2
  Path Command1 : InportShadow
  Position Error : Subsystem
  X pos PID : simulink/Continuous/PID Controller  Controller=PI  TimeDomain=Continuous-time  SampleTime=-1  IntegratorMethod=Forward Euler  FilterMethod=Forward Euler  Form=Parallel  UseFilter=on  ControllerParametersSource=internal  P=2  I=1.1  D=0  N=2.38928974494516  InitialConditionSource=internal  InitialConditionForIntegrator=0  InitialConditionForFilter=0  ExternalReset=none  LimitOutput=on  UpperSaturationLimit=2  LowerSaturationLimit=-2  LinearizeAsGain=on  AntiWindupMode=clamping  Kb=1  TrackingMode=off  Kt=1  PParamMin=[]  PParamMax=[]  IParamMin=[]  IParamMax=[]  DParamMin=[]  DParamMax=[]  NParamMin=[]  NParamMax=[]  KbParamMin=[]  KbParamMax=[]  KtParamMin=[]  KtParamMax=[]  POutMin=[]  POutMax=[]  IOutMin=[]  IOutMax=[]  DOutMin=[]  DOutMax=[]  NOutMin=[]  NOutMax=[]  KbOutMin=[]  KbOutMax=[]  KtOutMin=[]  KtOutMax=[]  IntegratorOutMin=[]  IntegratorOutMax=[]  FilterOutMin=[]  FilterOutMax=[]  SumOutMin=[]  SumOutMax=[]  SumI1OutMin=[]  SumI1OutMax=[]  SumI2OutMin=[]  SumI2OutMax=[]  SumI3OutMin=[]  SumI3OutMax=[]  SumDOutMin=[]  SumDOutMax=[]  SaturationOutMin=[]  SaturationOutMax=[]  IntegratorContinuousStateAttributes=''  IntegratorStateMustResolveToSignalObject=off  IntegratorRTWStateStorageClass=Auto  FilterContinuousStateAttributes=''  FilterStateMustResolveToSignalObject=off  FilterRTWStateStorageClass=Auto  DifferentiatorICPrevScaledInput=0  DifferentiatorOutMin=[]  DifferentiatorOutMax=[]  InitialConditionSetting=State (most efficient)  FilterDiffOutCoefMin=[]  FilterDiffOutCoefMax=[]  SumDenOutMin=[]  SumDenOutMax=[]  SumNumOutMin=[]  SumNumOutMax=[]  ReciprocalOutMin=[]  ReciprocalOutMax=[]  DivideOutMin=[]  DivideOutMax=[]  TunerSelectOption=Transfer Function Based (PID Tuner App)
  Y pos PID : simulink/Continuous/PID Controller  Controller=PI  TimeDomain=Continuous-time  SampleTime=-1  IntegratorMethod=Forward Euler  FilterMethod=Forward Euler  Form=Parallel  UseFilter=on  ControllerParametersSource=internal  P=2  I=1.1  D=0  N=0.5  InitialConditionSource=internal  InitialConditionForIntegrator=0  InitialConditionForFilter=0  ExternalReset=none  LimitOutput=on  UpperSaturationLimit=2  LowerSaturationLimit=-2  LinearizeAsGain=on  AntiWindupMode=none  Kb=1  TrackingMode=off  Kt=1  PParamMin=[]  PParamMax=[]  IParamMin=[]  IParamMax=[]  DParamMin=[]  DParamMax=[]  NParamMin=[]  NParamMax=[]  KbParamMin=[]  KbParamMax=[]  KtParamMin=[]  KtParamMax=[]  POutMin=[]  POutMax=[]  IOutMin=[]  IOutMax=[]  DOutMin=[]  DOutMax=[]  NOutMin=[]  NOutMax=[]  KbOutMin=[]  KbOutMax=[]  KtOutMin=[]  KtOutMax=[]  IntegratorOutMin=[]  IntegratorOutMax=[]  FilterOutMin=[]  FilterOutMax=[]  SumOutMin=[]  SumOutMax=[]  SumI1OutMin=[]  SumI1OutMax=[]  SumI2OutMin=[]  SumI2OutMax=[]  SumI3OutMin=[]  SumI3OutMax=[]  SumDOutMin=[]  SumDOutMax=[]  SaturationOutMin=[]  SaturationOutMax=[]  IntegratorContinuousStateAttributes=''  IntegratorStateMustResolveToSignalObject=off  IntegratorRTWStateStorageClass=Auto  FilterContinuousStateAttributes=''  FilterStateMustResolveToSignalObject=off  FilterRTWStateStorageClass=Auto  DifferentiatorICPrevScaledInput=0  DifferentiatorOutMin=[]  DifferentiatorOutMax=[]  InitialConditionSetting=State (most efficient)  FilterDiffOutCoefMin=[]  FilterDiffOutCoefMax=[]  SumDenOutMin=[]  SumDenOutMax=[]  SumNumOutMin=[]  SumNumOutMax=[]  ReciprocalOutMin=[]  ReciprocalOutMax=[]  DivideOutMin=[]  DivideOutMax=[]  TunerSelectOption=Transfer Function Based (PID Tuner App)
  Vy_cmd : Outport
  Vx_cmd : Outport  Port=2
  Path_cmd : Outport  Port=3
  tag scope: X_error=global, Y_error=global
  wires:
  Position Error/1(Y Error in Body Frame) -> [Y_error], Y pos PID/1  "Y error"
  Path Command/1 -> Position Error/1(Patch Command)
  State input/1 -> Position Error/2(State input)
  Position Error/2(X Error in body Frame) -> [X_error], X pos PID/1  "X error"
  X pos PID/1 -> Vx_cmd/1
  Path Command1/1 -> Path_cmd/1
  Y pos PID/1 -> Vy_cmd/1

== system UAV_USV_Simulator/High Level Controller/Cascaded PID/Velocity Controller ==
  Vy_cmd : Inport
  Vx_cmd : Inport  Port=2
  Path command : Inport  Port=3
  "State input " : Inport  Port=4
  Bus Creator1 : BusCreator  Inputs=4
  Bus Selector : BusSelector  OutputSignals=Psi_cmd,Alt_cmd
  Phi Command Control : Subsystem
  Theta Command Control : Subsystem
  Attitude Cmd : Outport
  wires:
  Bus Creator1/1 -> Attitude Cmd/1
  Bus Selector/2 -> Bus Creator1/4  "<Alt_cmd>"
  Theta Command Control/1(The_cmd) -> Bus Creator1/2  "The_cmd"
  Phi Command Control/1(Phi_cmd) -> Bus Creator1/1  "Phi_cmd"
  Bus Selector/1 -> Bus Creator1/3  "<Psi_cmd>"
  "State input "/1 -> Phi Command Control/2(Yb Velocity), Theta Command Control/2(Xb Velocity)
  Vy_cmd/1 -> Phi Command Control/1(Desired Yb Velocity)
  Path command/1 -> Bus Selector/1
  Vx_cmd/1 -> Theta Command Control/1(Desired Xb Velocity)

== system UAV_USV_Simulator/High Level Controller/Inverse kinematics architecture/Altitude Control ==
  Attitude Comand : Inport
  Z : Inport  Port=2
  Bus Selector : BusSelector  OutputSignals=Alt_cmd
  Bus Selector1 : BusSelector  OutputSignals=Z
  PID Controller : simulink/Continuous/PID Controller  Controller=PID  TimeDomain=Continuous-time  SampleTime=-1  IntegratorMethod=Forward Euler  FilterMethod=Forward Euler  Form=Parallel  UseFilter=on  ControllerParametersSource=internal  P=10  I=10  D=3  N=40  InitialConditionSource=internal  InitialConditionForIntegrator=4.35  InitialConditionForFilter=0  ExternalReset=none  ZeroCross=off  LimitOutput=on  UpperSaturationLimit=7  LowerSaturationLimit=2  LinearizeAsGain=on  AntiWindupMode=clamping  Kb=1  TrackingMode=off  Kt=1  PParamMin=[]  PParamMax=[]  IParamMin=[]  IParamMax=[]  DParamMin=[]  DParamMax=[]  NParamMin=[]  NParamMax=[]  KbParamMin=[]  KbParamMax=[]  KtParamMin=[]  KtParamMax=[]  POutMin=[]  POutMax=[]  IOutMin=[]  IOutMax=[]  DOutMin=[]  DOutMax=[]  NOutMin=[]  NOutMax=[]  KbOutMin=[]  KbOutMax=[]  KtOutMin=[]  KtOutMax=[]  IntegratorOutMin=[]  IntegratorOutMax=[]  FilterOutMin=[]  FilterOutMax=[]  SumOutMin=[]  SumOutMax=[]  SumI1OutMin=[]  SumI1OutMax=[]  SumI2OutMin=[]  SumI2OutMax=[]  SumI3OutMin=[]  SumI3OutMax=[]  SumDOutMin=[]  SumDOutMax=[]  SaturationOutMin=[]  SaturationOutMax=[]  IntegratorContinuousStateAttributes=''  IntegratorStateMustResolveToSignalObject=off  IntegratorRTWStateStorageClass=Auto  FilterContinuousStateAttributes=''  FilterStateMustResolveToSignalObject=off  FilterRTWStateStorageClass=Auto  DifferentiatorICPrevScaledInput=0  DifferentiatorOutMin=[]  DifferentiatorOutMax=[]  InitialConditionSetting=State (most efficient)  FilterDiffOutCoefMin=[]  FilterDiffOutCoefMax=[]  SumDenOutMin=[]  SumDenOutMax=[]  SumNumOutMin=[]  SumNumOutMax=[]  ReciprocalOutMin=[]  ReciprocalOutMax=[]  DivideOutMin=[]  DivideOutMax=[]  TunerSelectOption=Transfer Function Based (PID Tuner App)
  Sum : Sum  Inputs=|+-
  Out1 : Outport
  tag scope: Alt=global, Alt_PID=global, Alt_cmd=global, Alt_err=global
  wires:
  Attitude Comand/1 -> Bus Selector/1
  Bus Selector/1 -> Sum/1, [Alt_cmd]  "<Alt_cmd>"
  Sum/1 -> [Alt_err], PID Controller/1
  Z/1 -> Bus Selector1/1
  Bus Selector1/1 -> [Alt], Sum/2  "<Z>"
  PID Controller/1 -> Out1/1, [Alt_PID]

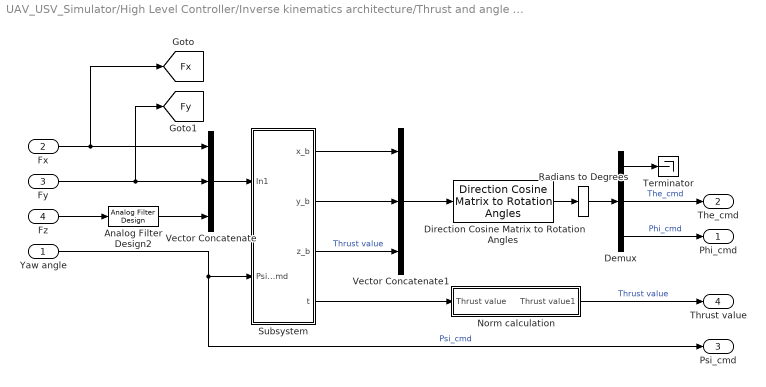
== system UAV_USV_Simulator/High Level Controller/Inverse kinematics architecture/Thrust and angle calculation3 ==
  Yaw angle : Inport
  Fx : Inport  Port=2
  Fy : Inport  Port=3
  Fz : Inport  Port=4
  Analog Filter Design2 : dsparch4/Analog Filter Design  method=Butterworth  filttype=Lowpass  N=15  Wlo=20*2*pi  Whi=80  Rp=2  Rs=40
  Demux : Demux  Outputs=3
  Direction Cosine Matrix to Rotation Angles : sharedtransform/Direction Cosine Matrix to Rotation Angles  rotationOrder=ZYX
      settings: SourceProductName=Aerospace Blockset  SourceProductBaseCode=AE
  Norm calculation : Subsystem
  Radians to Degrees : simulink_extras/Transformations/Radians to Degrees
  Subsystem : Subsystem
  Terminator : Terminator
  Vector Concatenate : Concatenate  NumInputs=3
  Vector Concatenate1 : Concatenate  NumInputs=3  Mode=Multidimensional array  ConcatenateDimension=2
  Phi_cmd : Outport
  The_cmd : Outport  Port=2
  Psi_cmd : Outport  Port=3
  Thrust value : Outport  Port=4
  tag scope: Fx=global, Fy=global
  wires:
  Demux/3 -> Phi_cmd/1  "Phi_cmd"
  Yaw angle/1 -> Psi_cmd/1, Subsystem/2(Psi_cmd)  "Psi_cmd"
  Subsystem/3(z_b) -> Vector Concatenate1/3  "Thrust value"
  Fx/1 -> [Fx], Vector Concatenate/1
  Vector Concatenate/1 -> Subsystem/1(In1)
  Subsystem/1(x_b) -> Vector Concatenate1/1
  Subsystem/2(y_b) -> Vector Concatenate1/2
  Vector Concatenate1/1 -> Direction Cosine Matrix to Rotation Angles/1
  Fz/1 -> Analog Filter Design2/1
  Fy/1 -> [Fy], Vector Concatenate/2
  Direction Cosine Matrix to Rotation Angles/1 -> Radians to Degrees/1
  Demux/1 -> Terminator/1
  Norm calculation/1(Thrust value1) -> Thrust value/1  "Thrust value"
  Subsystem/4(t) -> Norm calculation/1(Thrust value)
  Radians to Degrees/1 -> Demux/1
  Analog Filter Design2/1 -> Vector Concatenate/3
  Demux/2 -> The_cmd/1  "The_cmd"

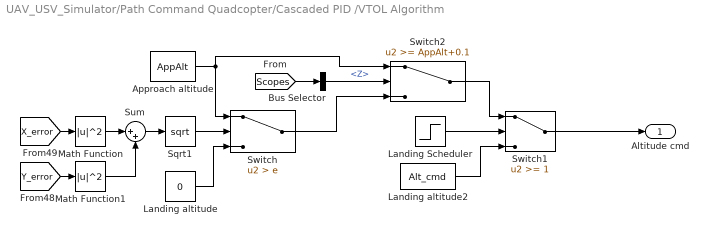
== system UAV_USV_Simulator/Path Command Quadcopter/Cascaded PID /VTOL Algorithm ==
  Approach altitude : Constant  Value=AppAlt
  Bus Selector : BusSelector  OutputSignals=Z
  Landing altitude2 : Constant  Value=Alt_cmd
  Landing altitude : Constant  Value=0
  Landing Scheduler : Step  Time=LandingSchedule  After=EnableVTOL  SampleTime=0
  Math Function : Math  Operator=magnitude^2  SaturateOnIntegerOverflow=on
  Math Function1 : Math  Operator=magnitude^2  SaturateOnIntegerOverflow=on
  Sqrt1 : Sqrt  SaturateOnIntegerOverflow=on
  Sum : Sum  Inputs=|++
  Switch : Switch  Criteria=u2 > Threshold  Threshold=e
  Switch1 : Switch  Threshold=1
  Switch2 : Switch  Threshold=AppAlt+0.1
  Altitude cmd : Outport
  wires:
  Landing altitude2/1 -> Switch1/3
  Landing Scheduler/1 -> Switch1/2
  Switch1/1 -> Altitude cmd/1
  Math Function/1 -> Sum/1
  [X_error] -> Math Function/1
  Sum/1 -> Sqrt1/1
  Sqrt1/1 -> Switch/2
  [Y_error] -> Math Function1/1
  Math Function1/1 -> Sum/2
  Switch2/1 -> Switch1/1
  Bus Selector/1 -> Switch2/2  "<Z>"
  Switch/1 -> Switch2/3
  Landing altitude/1 -> Switch/3
  Approach altitude/1 -> Switch/1, Switch2/1
  [Scopes] -> Bus Selector/1

== system UAV_USV_Simulator/Path Command Quadcopter/Inverse Kinematics/Signal Builder ==
  Demux : Demux  Tag=STV Demux  Outputs=3
  FromWs : FromWorkspace  Tag=STV FromWs  VariableName=tuvar  SampleTime=0
      SigBuilderData=|
      | common.afterFinalStr = 'Extrapolate'
      | common.sampleTime = 0
      | dataSet.timeRange = [0 20]
      | dataSet.name = 'Imported_Group 1'
      | sbobj.Groups.Name = 'Imported_Group 1'
      | sbobj.Groups.Signals(1).Name = 'T1'
      | sbobj.Groups.Signals(1).XData = [0 0.0100050025013 0.0200100050025 0.0300150075038 0.040020010005 0.0500250125063 0.0600300150075 0.0700350175088 0.08004002001 0.0900450225113 0.100050025013 0.110055027514 ... (2000 elements, 1x2000)]
      | sbobj.Groups.Signals(1).YData = [1.00150059799e-07 7.10305434067e-06 2.12396351659e-05 4.26638794652e-05 7.15535255738e-05 0.000108109990893 0.000152557599906 0.000205142070924 0.000266128287292 0.00033579745796 0.00041444385252 0.000502371363491 ... (2000 elements, 1x2000)]
      | sbobj.Groups.Signals(2).Name = 'T7'
      | sbobj.Groups.Signals(2).XData = [0 0.0100050025013 0.0200100050025 0.0300150075038 0.040020010005 0.0500250125063 0.0600300150075 0.0700350175088 0.08004002001 0.0900450225113 0.100050025013 0.110055027514 ... (2000 elements, 1x2000)]
      | sbobj.Groups.Signals(2).YData = [0 0.000700290428087 0.00141365808252 0.00214242442993 0.00288896461086 0.00365564653192 0.00444476090128 0.00525844710185 0.00609862163676 0.00696691706677 0.007864639456 0.00879275109708 ... (2000 elements, 1x2000)]
      | sbobj.Groups.Signals(3).Name = 'T13'
      | sbobj.Groups.Signals(3).XData = [0 0.0100050025013 0.0200100050025 0.0300150075038 0.040020010005 0.0500250125063 0.0600300150075 0.0700350175088 0.08004002001 0.0900450225113 0.100050025013 0.110055027514 ... (2000 elements, 1x2000)]
      | sbobj.Groups.Signals(3).YData = [0.0700290428087 0.0713367654436 0.0728766347404 0.0746540180937 0.0766681921054 0.0789114369362 0.0813686200575 0.0840174534907 0.0868295430012 0.0897722389222 0.0928111641082 0.0959131650763 ... (2000 elements, 1x2000)]
      | sbobj.Groups.TimeRange = [0 20]
  T1 : Outport  Tag=STV Outport
  T7 : Outport  Tag=STV Outport  Port=2
  T13 : Outport  Tag=STV Outport  Port=3
  wires:
  Demux/1 -> T1/1
  FromWs/1 -> Demux/1
  Demux/2 -> T7/1
  Demux/3 -> T13/1

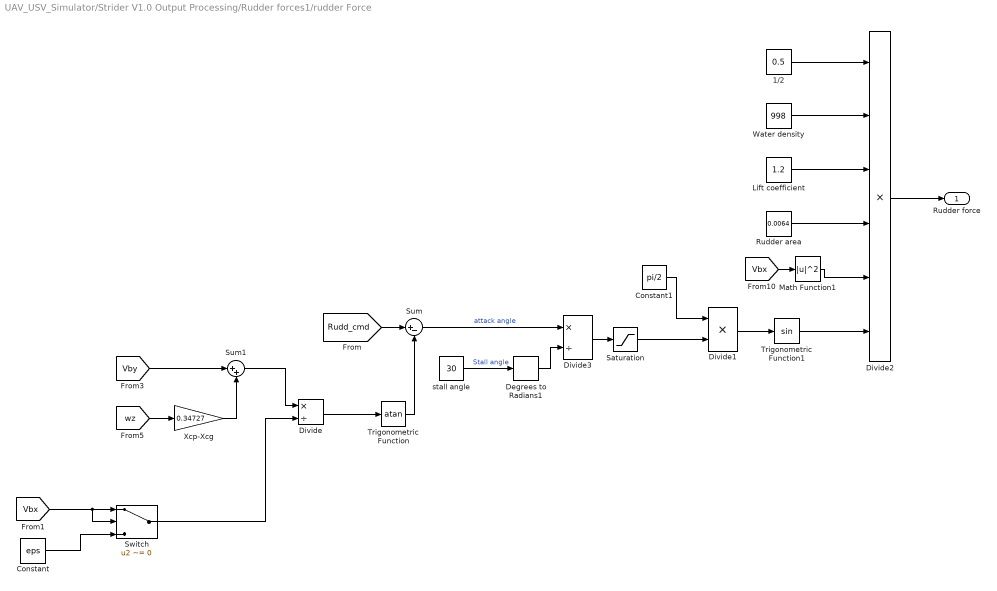
== system UAV_USV_Simulator/Strider V1.0 Output Processing/Rudder forces1/rudder Force  ==
  1/2 : Constant  Value=0.5
  Constant : Constant  Value=eps
  Constant1 : Constant  Value=pi/2
  Degrees to Radians1 : simulink_extras/Transformations/Degrees to Radians
  Divide : Product  Inputs=*/
  Divide1 : Product  Inputs=**
  Divide2 : Product  Inputs=******
  Divide3 : Product  Inputs=*/
  Lift coefficient : Constant  Value=1.2
  Math Function1 : Math  Operator=magnitude^2  SaturateOnIntegerOverflow=on
  Rudder area : Constant  Value=0.0064
  Saturation : Saturate  UpperLimit=1  LowerLimit=-1
  Sum : Sum  Inputs=|+-
  Sum1 : Sum  Inputs=|++
  Switch : Switch  Criteria=u2 ~= 0
  Trigonometric Function : Trigonometry  Operator=atan
  Trigonometric Function1 : Trigonometry
  Water density : Constant  Value=998
  Xcp-Xcg : Gain  Gain=0.34727
  stall angle : Constant  Value=30
  Rudder force : Outport
  wires:
  Divide2/1 -> Rudder force/1
  Water density/1 -> Divide2/2
  [Vbx] -> Math Function1/1
  Sum1/1 -> Divide/1
  Rudder area/1 -> Divide2/4
  1/2/1 -> Divide2/1
  Lift coefficient/1 -> Divide2/3
  Constant1/1 -> Divide1/1
  Math Function1/1 -> Divide2/5
  Trigonometric Function1/1 -> Divide2/6
  [Rudd_cmd] -> Sum/1
  [wz] -> Xcp-Xcg/1
  Trigonometric Function/1 -> Sum/2
  [Vby] -> Sum1/1
  Divide1/1 -> Trigonometric Function1/1
  Xcp-Xcg/1 -> Sum1/2
  Sum/1 -> Divide3/1  "attack angle"
  stall angle/1 -> Degrees to Radians1/1  "Stall angle"
  Divide3/1 -> Saturation/1
  Saturation/1 -> Divide1/2
  Divide/1 -> Trigonometric Function/1
  Degrees to Radians1/1 -> Divide3/2
  [Vbx] -> Switch/2, Switch/1
  Constant/1 -> Switch/3
  Switch/1 -> Divide/2

== system UAV_USV_Simulator/Attitude Controller/Altitude Control/Altitude controller/Altitude PID Control ==
  Alt_cmd : Inport
  Z : Inport  Port=2
  Bus Selector : BusSelector  OutputSignals=Alt_cmd
  PID Controller : simulink/Continuous/PID Controller  Controller=PID  TimeDomain=Continuous-time  SampleTime=-1  IntegratorMethod=Forward Euler  FilterMethod=Forward Euler  Form=Parallel  UseFilter=on  ControllerParametersSource=internal  P=170.242040782586  I=28.86184465251  D=50  N=50  InitialConditionSource=internal  InitialConditionForIntegrator=0  InitialConditionForFilter=0  ExternalReset=none  ZeroCross=off  LimitOutput=on  UpperSaturationLimit=90  LowerSaturationLimit=35  LinearizeAsGain=on  AntiWindupMode=clamping  Kb=1  TrackingMode=off  Kt=1  PParamMin=[]  PParamMax=[]  IParamMin=[]  IParamMax=[]  DParamMin=[]  DParamMax=[]  NParamMin=[]  NParamMax=[]  KbParamMin=[]  KbParamMax=[]  KtParamMin=[]  KtParamMax=[]  POutMin=[]  POutMax=[]  IOutMin=[]  IOutMax=[]  DOutMin=[]  DOutMax=[]  NOutMin=[]  NOutMax=[]  KbOutMin=[]  KbOutMax=[]  KtOutMin=[]  KtOutMax=[]  IntegratorOutMin=[]  IntegratorOutMax=[]  FilterOutMin=[]  FilterOutMax=[]  SumOutMin=[]  SumOutMax=[]  SumI1OutMin=[]  SumI1OutMax=[]  SumI2OutMin=[]  SumI2OutMax=[]  SumI3OutMin=[]  SumI3OutMax=[]  SumDOutMin=[]  SumDOutMax=[]  SaturationOutMin=[]  SaturationOutMax=[]  IntegratorContinuousStateAttributes=''  IntegratorStateMustResolveToSignalObject=off  IntegratorRTWStateStorageClass=Auto  FilterContinuousStateAttributes=''  FilterStateMustResolveToSignalObject=off  FilterRTWStateStorageClass=Auto  DifferentiatorICPrevScaledInput=0  DifferentiatorOutMin=[]  DifferentiatorOutMax=[]  InitialConditionSetting=State (most efficient)  FilterDiffOutCoefMin=[]  FilterDiffOutCoefMax=[]  SumDenOutMin=[]  SumDenOutMax=[]  SumNumOutMin=[]  SumNumOutMax=[]  ReciprocalOutMin=[]  ReciprocalOutMax=[]  DivideOutMin=[]  DivideOutMax=[]  TunerSelectOption=Transfer Function Based (PID Tuner App)
  Sum : Sum  Inputs=|+-
  Out : Outport
  wires:
  Alt_cmd/1 -> Bus Selector/1
  Bus Selector/1 -> Sum/1  "<Alt_cmd>"
  PID Controller/1 -> Out/1
  Sum/1 -> PID Controller/1
  Z/1 -> Sum/2
